simulink library "SplineInt"  (Simulink 7.9)
settings: Solver=ode45  StartTime=0.0  StopTime=10.0  RelTol=1e-3
libraries: dspsigops x1
settings Model: Creator=Mihail  LastModifiedBy=Mihail

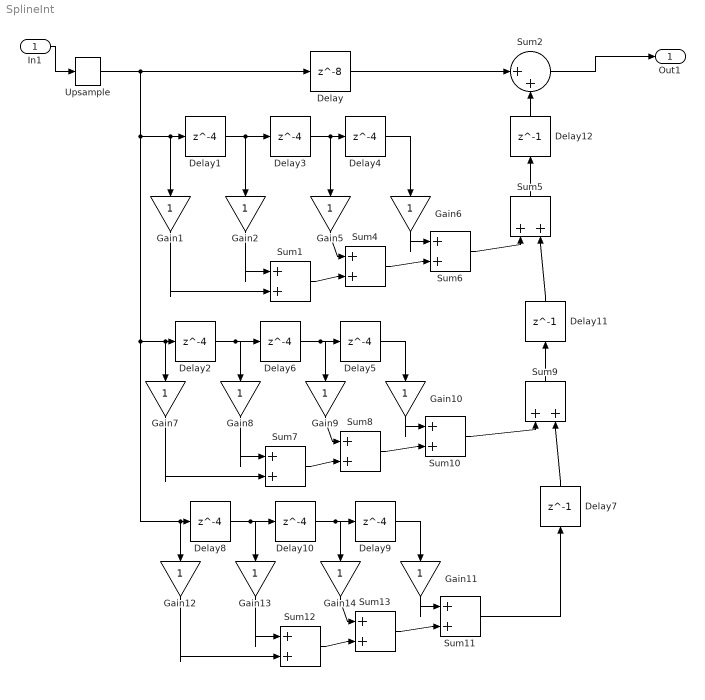
== system SplineInt ==
  In1 : Inport
  Delay : Delay  DelayLength=8
  Delay{1..6,8..10} (9 alike) : Delay  DelayLength=4
  Delay11 : Delay  DelayLength=1
  Delay12 : Delay  DelayLength=1
  Delay7 : Delay  DelayLength=1
  Gain{1..2,5..14} (12 alike) : Gain  RndMeth=Convergent
  Sum{1..2,4..13} (12 alike) : Sum  Inputs=|++  SaturateOnIntegerOverflow=on
  Upsample : dspsigops/Upsample  N=4  phase=0  InputProcessing=Columns as channels (frame based)  RateOptions=Enforce single-rate processing  ic=0  mode=Unused parameter value
  Out1 : Outport
  wires:
  In1/1 -> Upsample/1
  Upsample/1 -> Delay/1, Delay1/1, Gain1/1, Delay2/1, Gain7/1, Delay8/1, Gain12/1
  Delay1/1 -> Delay3/1, Gain2/1
  Delay3/1 -> Delay4/1, Gain5/1
  Delay4/1 -> Gain6/1
  Gain1/1 -> Sum1/2
  Gain2/1 -> Sum1/1
  Sum1/1 -> Sum4/2
  Gain5/1 -> Sum4/1
  Sum4/1 -> Sum6/2
  Gain6/1 -> Sum6/1
  Sum6/1 -> Sum5/1
  Delay2/1 -> Delay6/1, Gain8/1
  Delay6/1 -> Delay5/1, Gain9/1
  Gain7/1 -> Sum7/2
  Gain8/1 -> Sum7/1
  Sum7/1 -> Sum8/2
  Gain9/1 -> Sum8/1
  Sum8/1 -> Sum10/2
  Gain10/1 -> Sum10/1
  Sum10/1 -> Sum9/1
  Delay5/1 -> Gain10/1
  Delay8/1 -> Delay10/1, Gain13/1
  Delay10/1 -> Delay9/1, Gain14/1
  Gain12/1 -> Sum12/2
  Gain13/1 -> Sum12/1
  Sum12/1 -> Sum13/2
  Gain14/1 -> Sum13/1
  Sum13/1 -> Sum11/2
  Gain11/1 -> Sum11/1
  Delay9/1 -> Gain11/1
  Delay7/1 -> Sum9/2
  Sum11/1 -> Delay7/1
  Sum9/1 -> Delay11/1
  Delay11/1 -> Sum5/2
  Delay/1 -> Sum2/1
  Delay12/1 -> Sum2/2
  Sum5/1 -> Delay12/1
  Sum2/1 -> Out1/1
